simulink model "FOC_beautified"  (R2022b)
settings: Solver=ode1  StartTime=0.0  StopTime=0.2  FixedStep=ctrlConst.TsSwitch  MaxStep=1e-6  RelTol=1e-3  EnableMultiTasking=on
undefined symbols (not defined in the file): ECM, f32_P_AngleCompCur, f32_P_AngleCompVol, f32_P_Coef, f32_P_IdInIF_A, f32_P_Modulation, FFW_enable, g_msgCore0to2_AcrKi, g_msgCore0to2_AcrKiStb, g_msgCore0to2_AcrKp, g_msgCore0to2_AcrKpStb, g_msgCore0to2_AcrSwtHiRpm, g_msgCore0to2_AcrSwtLoRpm, g_msgCore0to2_AfrKp, g_msgCore0to2_AfrTi, g_msgCore0to2_arc_dd_fi, g_msgCore0to2_CalibEn, g_msgCore0to2_clpwitch, g_msgCore0to2_DecoupleEn, g_msgCore0to2_dqLpf, g_msgCore0to2_dqLpfSpdCoef, g_msgCore0to2_FFW_Gain, g_msgCore0to2_linearKpEn, g_msgCore0to2_maxCur, g_msgCore0to2_maxFwcCurRatio, g_msgCore0to2_motorseq, g_msgCore0to2_MTPA_Gain, g_msgCore0to2_pwmFrqSet, g_msgCore0to2_spdswitch, IdROL_C, PWMFrqSwitch_C, SC_Ld_P, SC_Lq_P, SC_Psi_P, Tsw, u16_P_MotorPair
libraries: MathLib x6, simulink x1
(part 1 of 2)
settings Model: Creator=M00039784  LastModifiedBy=HP
settings SolverCC: AlgebraicLoopSolver=TrustRegion  InsertRTBMode=Never (minimum delay)
settings DataIOCC: LimitDataPoints=on  SaveFormat=Array  SaveOutput=off  SaveTime=off
settings OptimizationCC: DefaultParameterBehavior=Inlined  UseDivisionForNetSlopeComputation=on  UseFloatMulNetSlope=on  DefaultUnderspecifiedDataType=single  InlineInvariantSignals=on  PassReuseOutputArgsAs=Individual arguments  ExpressionDepthLimit=2147483647  ZeroExternalMemoryAtStartup=off  ZeroInternalMemoryAtStartup=off  NoFixptDivByZeroProtection=on  EfficientFloat2IntCast=on  LifeSpan=1  EfficientTunableParamExpr=on
settings DebuggingCC: ReadBeforeWriteMsg=DisableAll  WriteAfterWriteMsg=DisableAll  WriteAfterReadMsg=DisableAll  AlgebraicLoopMsg=none  MultiTaskDSMMsg=none  SingleTaskRateTransMsg=error  IntegerOverflowMsg=none  ParameterPrecisionLossMsg=none  FcnCallInpInsideContextMsg=warning  BusObjectLabelMismatch=none  AssertControl=DisableAll  AllowSymbolicDim=off  StateNameClashWarn=warning  SFUnexpectedBacktrackingDiag=warning  SFNoUnconditionalDefaultTransitionDiag=warning  SFExecutionAtInitializationDiag=none  SFMachineParentedDataDiag=warning  IntegerSaturationMsg=none  UnitsInconsistencyMsg=none  ArithmeticOperatorsInVariantConditions=warning
settings HardwareCC: ProdBitPerPointer=32  ProdBitPerSizeT=32  ProdBitPerPtrDiffT=32  ProdLargestAtomicFloat=None  ProdWordSize=32  ProdHWDeviceType=Infineon->TriCore
settings ModelReferenceCC: UpdateModelReferenceTargets=IfOutOfDate  EnableRefExpFcnMdlSchedulingChecks=on  ModelReferenceNumInstancesAllowed=Single  PropagateSignalLabelsOutOfModel=off
settings SFSimCC: SFSimEcho=off  SimUseLocalCustomCode=off  SimGenImportedTypeDefs=on  MATLABDynamicMemAlloc=off  CustomCodeUndefinedFunction=UseInterfaceOnly
settings RTWCC: Description=Embedded Coder  SystemTargetFile=ert.tlc  GenCodeOnly=on  GenerateMakefile=off  TemplateMakefile=ec_target.tmf  RTWVerbose=off  RTWUseLocalCustomCode=off  CodeExecutionProfiling=on  CodeProfilingSaveOptions=AllData  CodeProfilingInstrumentation=detailed
settings CodeAppCC: ForceParamTrailComments=on  IgnoreCustomStorageClasses=off  IgnoreTestpoints=on  MaxIdLength=64  SimulinkDataObjDesc=on  MATLABFcnDesc=on  CustomSymbolStrGlobalVar=pmsmfoc_rt$N$M  CustomSymbolStrType=pmsmfoc_$N$M  CustomSymbolStrFcn=$N$M$F  CustomSymbolStrFcnArg=$I$N$M  CustomSymbolStrMacro=$N$M  InsertBlockDesc=on  StateflowObjectComments=on  MATLABSourceComments=on  InternalIdentifier=Classic
settings ERTTargetCC: TargetLangStandard=C99 (ISO)  UtilityFuncGeneration=Shared location  MultiwordLength=2048  CombineSignalStateStructs=on  SupportAbsoluteTime=off  SupportNonFinite=off  SupportComplex=off  SupportNonInlinedSFcns=on  RemoveResetFunc=off  ParenthesesLevel=Maximum  GenerateASAP2=on  InlinedParameterPlacement=NonHierarchical  ERTCustomFileTemplate=example_file_process.tlc  EnableDataOwnership=on  ConvertIfToSwitch=off  SuppressUnreachableDefaultCases=off  MemSecPackage=Simulink  MemSecDataConstants=MemConst  MemSecDataParameters=MemConstVolatile
settings ConfigComp: CovMetricSettings=dcmtrzow  CovHTMLOptions=-aTS=1 -bRG=1 -bTC=1 -hTR=0 -nFC=0 -scm=1 -bcm=1 -xEv=0  CovSaveCumulativeToWorkspaceVar=on  CovSaveSingleToWorkspaceVar=on  CovExternalEMLEnable=off  CovSFcnEnable=off
settings SimscapeCC: SimscapeNormalizeSystem=off

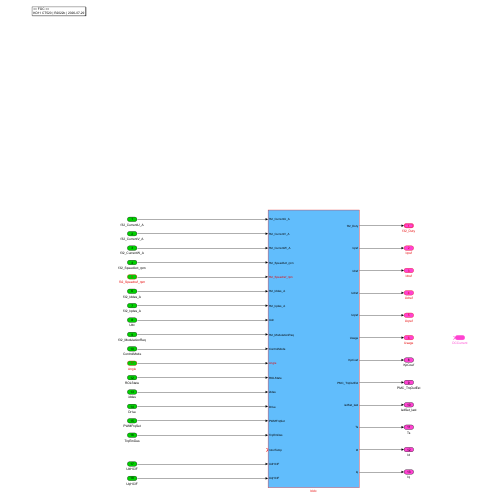
[thumbnail: Simulink's stored preview of the top-level diagram]
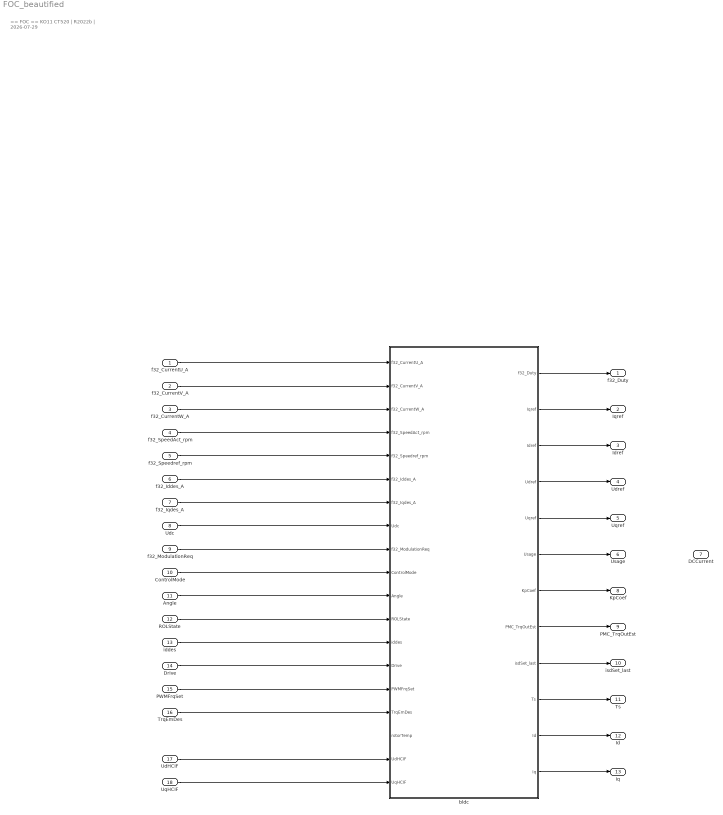
== system FOC_beautified ==
  note: == FOC ==
      | KO11 CT520 | R2022b | 2026-07-29
  f32_CurrentU_A : Inport  OutDataTypeStr=single  PortDimensions=1  SampleTime=0.0001
  f32_CurrentV_A : Inport  Port=2  OutDataTypeStr=single  PortDimensions=1  SampleTime=0.0001
  f32_CurrentW_A : Inport  Port=3  OutDataTypeStr=single  PortDimensions=1  SampleTime=0.0001
  f32_SpeedAct_rpm : Inport  Port=4  OutDataTypeStr=single  PortDimensions=1  SampleTime=0.0001
  f32_Speedref_rpm : Inport  Port=5  OutDataTypeStr=single  PortDimensions=1
  f32_Iddes_A : Inport  Port=6
  f32_Iqdes_A : Inport  Port=7
  "Udc " : Inport  Port=8  OutDataTypeStr=single  PortDimensions=1
  f32_ModulationReq : Inport  Port=9  OutDataTypeStr=single  PortDimensions=1
  ControlMode : Inport  Port=10  OutDataTypeStr=Enum: ECM  PortDimensions=1  SampleTime=0.0001
  Angle : Inport  Port=11  OutDataTypeStr=uint16  PortDimensions=1  SampleTime=0.0001
  ROLState : Inport  Port=12
  iddes : Inport  Port=13
  Drive : Inport  Port=14  OutDataTypeStr=boolean
  PWMFrqSet : Inport  Port=15
  TrqEmDes : Inport  Port=16
  UdHCIF : Inport  Port=17
  UqHCIF : Inport  Port=18
  bldc : Subsystem
  f32_Duty : Outport  OutDataTypeStr=Bus: Duty
  Iqref : Outport  Port=2
  Idref : Outport  Port=3
  Udref : Outport  Port=4
  Uqref : Outport  Port=5
  Usage : Outport  Port=6
  DCCurrent : Outport  Port=7
  KpCoef : Outport  Port=8
  PMC_TrqOutEst : Outport  Port=9
  isdSet_last : Outport  Port=10
  Ts : Outport  Port=11
  Id : Outport  Port=12
  Iq : Outport  Port=13
  wires:
  bldc/6(Usage) -> Usage/1
  f32_Speedref_rpm/1 -> bldc/5(f32_Speedref_rpm)
  f32_Iqdes_A/1 -> bldc/7(f32_Iqdes_A)
  bldc/2(Iqref) -> Iqref/1
  Angle/1 -> bldc/11(Angle)
  bldc/5(Uqref) -> Uqref/1
  f32_CurrentU_A/1 -> bldc/1(f32_CurrentU_A)
  ControlMode/1 -> bldc/10(ControlMode)
  bldc/3(Idref) -> Idref/1
  f32_ModulationReq/1 -> bldc/9(f32_ModulationReq)
  f32_CurrentV_A/1 -> bldc/2(f32_CurrentV_A)
  bldc/1(f32_Duty) -> f32_Duty/1
  f32_SpeedAct_rpm/1 -> bldc/4(f32_SpeedAct_rpm)
  f32_Iddes_A/1 -> bldc/6(f32_Iddes_A)
  f32_CurrentW_A/1 -> bldc/3(f32_CurrentW_A)
  "Udc "/1 -> bldc/8("Udc ")
  bldc/4(Udref) -> Udref/1
  ROLState/1 -> bldc/12(ROLState)
  iddes/1 -> bldc/13(iddes)
  Drive/1 -> bldc/14(Drive)
  PWMFrqSet/1 -> bldc/15(PWMFrqSet)
  bldc/7(KpCoef) -> KpCoef/1
  bldc/8(PMC_TrqOutEst) -> PMC_TrqOutEst/1
  TrqEmDes/1 -> bldc/16(TrqEmDes)
  bldc/9(isdSet_last) -> isdSet_last/1
  bldc/10(Ts) -> Ts/1
  bldc/11(Id) -> Id/1
  bldc/12(Iq) -> Iq/1
  UqHCIF/1 -> bldc/19(UqHCIF)
  UdHCIF/1 -> bldc/18(UdHCIF)

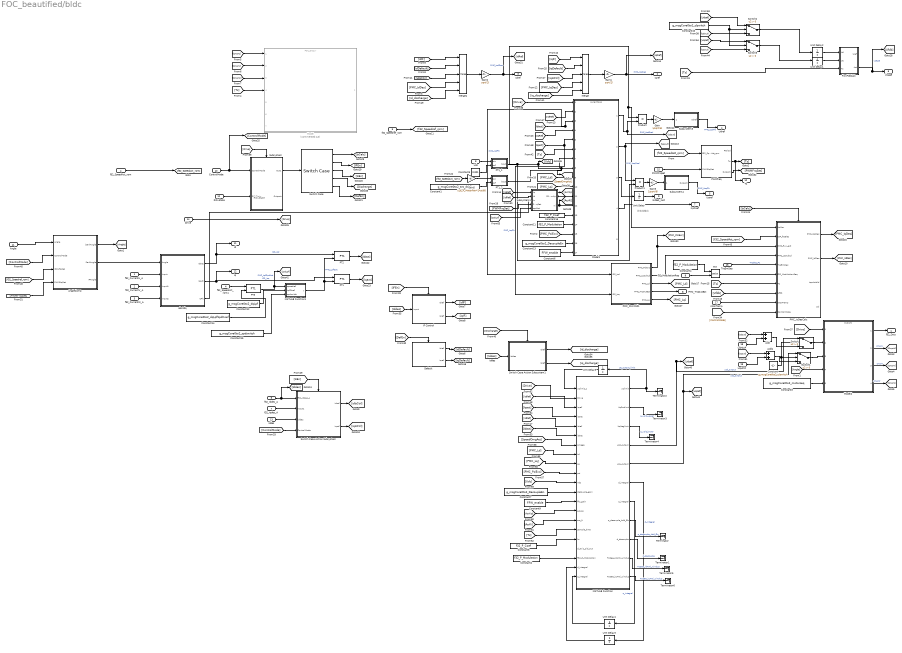
== system FOC_beautified/bldc ==
  note: ROLState
  note: 总电流输出
  f32_CurrentU_A : Inport  OutDataTypeStr=single  PortDimensions=1  SampleTime=0.0001
  f32_CurrentV_A : Inport  Port=2  OutDataTypeStr=single  PortDimensions=1  SampleTime=0.0001
  f32_CurrentW_A : Inport  Port=3  OutDataTypeStr=single  PortDimensions=1  SampleTime=0.0001
  f32_SpeedAct_rpm : Inport  Port=4  OutDataTypeStr=single  PortDimensions=1  SampleTime=0.0001
  f32_Speedref_rpm : Inport  Port=5  OutDataTypeStr=single  PortDimensions=1  SampleTime=0.0001
  f32_Iddes_A : Inport  Port=6
  f32_Iqdes_A : Inport  Port=7
  "Udc " : Inport  Port=8  OutDataTypeStr=single  PortDimensions=1
  f32_ModulationReq : Inport  Port=9
  ControlMode : Inport  Port=10  OutDataTypeStr=Enum: ECM  PortDimensions=1  SampleTime=0.0001
  Angle : Inport  Port=11  OutDataTypeStr=uint16  PortDimensions=1  SampleTime=0.0001
  ROLState : Inport  Port=12
  iddes : Inport  Port=13
  Drive : Inport  Port=14
  PWMFrqSet : Inport  Port=15
  TrqEmDes : Inport  Port=16
  rotorTemp : Inport  Port=17
  UdHCIF : Inport  Port=18
  UqHCIF : Inport  Port=19
  Add : Sum
  Add1 : Sum
  AngleComp : Subsystem  TreatAsAtomicUnit=on
  Constant : Constant  Value=g_msgCore0to2_clpwitch
  Constant1 : Constant  Value=g_msgCore0to2_arc_dd_fi  OutDataTypeStr=single
  Constant10 : Constant  Value=g_msgCore0to2_clpwitch
  Constant11 : Constant  Value=f32_P_Modulation
  Constant12 : Constant  Value=g_msgCore0to2_dqLpf
  Constant13 : Constant  Value=g_msgCore0to2_DecoupleEn
  Constant14 : Constant  Value=g_msgCore0to2_dqLpfSpdCoef
  Constant15 : Constant  Value=g_msgCore0to2_spdswitch
  Constant16 : Constant  Value=f32_P_Coef
  Constant2 : Constant  Value=f32_P_Modulation
  Constant3 : Constant  Value=g_msgCore0to2_motorseq  OutDataTypeStr=uint16
  Constant4 : Constant  Value=f32_P_Modulation  OutDataTypeStr=single
  Constant5 : Constant  Value=0.001  OutDataTypeStr=single
  Constant6 : Constant  Value=FFW_enable
  Constant7 : Constant  Value=g_msgCore0to2_DecoupleEn
  Constant8 : Constant  Value=f32_P_Coef
  Constant9 : Constant  Value=FFW_enable
  Default : Subsystem  TreatAsAtomicUnit=on
  FwcFdbCalc : Subsystem
  Gain : Gain  Gain=1/sqrt(6)
  Gain1 : Gain  Gain=sqrt(2)
  Gain2 : Gain  Gain=sqrt(2)
  Gain3 : Gain  Gain=1/sqrt(6)
  Gain5 : Gain  Gain=u16_P_MotorPair*2*pi/60
  IF Control : Subsystem  TreatAsAtomicUnit=on
  MATLAB Function : MATLAB Function  TreatAsAtomicUnit=on
  MATLAB Function1 : MATLAB Function  TreatAsAtomicUnit=on
  Merge : Merge  Inputs=5  InitialOutput=0
  Merge1 : Merge  Inputs=5  InitialOutput=0
  Min : MinMax  Inputs=2
  Model : ModelReference  Commented=on  ModelNameDialog=FOC_DCCur.slx  SimulationMode=Normal  ModelReferenceVersion=1.22
  Model1 : ModelReference  ModelNameDialog=currentloop.slxp  ModelReferenceVersion=1.125  CopyOfModelProtected=on
  Model2 : ModelReference  ModelNameDialog=SVPWM.slxp  ModelReferenceVersion=1.116  CopyOfModelProtected=on
  PMC_IsDesCalc : Subsystem
  PMC_PsmMdl1 : Subsystem
  PT1 : MathLib/PT1  SystemSampleTime=-1  VariantActivationTime=update diagram  Latency=0  AutoFrameSizeCalculation=off
  PT1_1 : Subsystem
  PT1_2 : Subsystem
  PT2 : MathLib/PT1  SystemSampleTime=-1  VariantActivationTime=update diagram  Latency=0  AutoFrameSizeCalculation=off
  PT3 : MathLib/PT1  SystemSampleTime=-1  VariantActivationTime=update diagram  Latency=0  AutoFrameSizeCalculation=off
  PWMfreq : Subsystem
  Product : Product
  Product1 : Product
  Subsystem : Subsystem
  Subsystem1 : Subsystem
  Subsystem3 : Subsystem
  Subsystem4 : Subsystem
  Switch{,1..3} (4 alike) : Switch  Criteria=u2 > Threshold  SaturateOnIntegerOverflow=off  InputSameDT=off
  Switch Case : SwitchCase  CaseConditions={[ECM.nCtrl,ECM.TrqCtrl],ECM.IFCtrl,[ECM.IsCtrl,ECM.alOfsCal],ECM.Discharge}
  Switch Case Action Subsystem : Subsystem  TreatAsAtomicUnit=on
  Switch Case Action Subsystem1 : Subsystem  TreatAsAtomicUnit=on
  Terminator{,1..6} (7 alike) : Terminator
  Unit Delay{,1..5} (6 alike) : UnitDelay  SampleTime=-1  HasFrameUpgradeWarning=on
  abc2dq : Subsystem
  f32_SpeedAct_rpm1 : InportShadow  Port=4  OutDataTypeStr=single  PortDimensions=1  SampleTime=0.0001
  f32_Duty : Outport  OutDataTypeStr=Bus: Duty
  Iqref : Outport  Port=2
  Idref : Outport  Port=3
  Udref : Outport  Port=4
  Uqref : Outport  Port=5
  Usage : Outport  Port=6
  KpCoef : Outport  Port=7
  PMC_TrqOutEst : Outport  Port=8
  isdSet_last : Outport  Port=9
  Ts : Outport  Port=10
  Id : Outport  Port=11
  Iq : Outport  Port=12
  wires:
  Model2/1 -> f32_Duty/1
  Model1/1 -> Product/2, [Udout]  "PMC_UsdScal"
  f32_SpeedAct_rpm/1 -> [f32_SpeedAct_rpm]
  Model1/2 -> Product1/1, [Uqout]  "PMC_UsqScal"
  PWMfreq/2(Ts) -> Ts/1, [Ts]
  [f32_SpeedAct_rpm] -> PWMfreq/1(f32_SpeedAct_rpm)
  ControlMode/1 -> [ControlMode], Subsystem/1(ControlMode)
  AngleComp/1(iparkAngle) -> [Angle]
  [Idact] -> Model1/3, PMC_PsmMdl1/1(ISP_Isd)  "PMC_isdFlt"
  PT1_1/1(bout) -> Product/1, PMC_IsDesCalc/1(UsMax), [Udc], Model1/7, Product1/2
  [Iqact] -> PMC_PsmMdl1/2(ISP_Isq), Model1/5  "PMC_isqFlt"
  [Ts] -> Model/4
  Model2/2 -> [CmprU]  "cmprU"
  Model2/3 -> [CmprV]  "cmprV"
  Model2/4 -> [CmprW]  "cmprW"
  [CmprW] -> Model/3
  [CmprV] -> Model/2
  [CmprU] -> Model/1
  f32_Iddes_A/1 -> [Iddes], Switch Case Action Subsystem/1(f32_Iddes_A)
  f32_Iqdes_A/1 -> Switch Case Action Subsystem/2(Input1)
  Default/1("Idref ") -> [idDefault]
  [idDefault] -> Merge1/2
  IF Control/1(Idref) -> [idIF]
  [idIF] -> Merge1/1
  IF Control/2(Iqref) -> [iqIF]
  Switch Case Action Subsystem/1("Idref ") -> [idIsCtrl]
  [idIsCtrl] -> Merge1/3
  Merge/1 -> Gain1/1
  [IqRef] -> Model1/4
  Default/2(Iqref) -> [iqDefault]
  Switch Case Action Subsystem/2(Iqref) -> [iqIsCtrl]
  [IFEn] -> IF Control/Action
  Switch Case/2 -> [IFEn]
  [IsEn] -> Switch Case Action Subsystem/Action
  Switch Case/3 -> [IsEn]
  Switch Case/5 -> [DefEn]
  [DefEn] -> Default/Action
  Subsystem/1(Out1) -> Switch Case/1
  ROLState/1 -> Subsystem/2(ROLState)
  iddes/1 -> Switch Case Action Subsystem/3(iddes)
  [ControlMode] -> Switch Case Action Subsystem/4(ControlMode)
  [Iddes] -> IF Control/1(Input)
  Drive/1 -> [Drive]
  [Drive] -> Model1/1
  [Drive] -> Model2/1
  [f32_SpeedAct_rpm] -> Gain5/1
  [Drive] -> Subsystem/Enable
  Model1/3 -> Unit Delay/1
  Unit Delay/1 -> isdSet_last/1
  [Ts] -> Model1/6
  PWMFrqSet/1 -> PWMfreq/2(PWMFrqSet)
  Gain1/1 -> [IqRef], Iqref/1  "PMC_IsqDes"
  Model1/4 -> KpCoef/1
  Product/1 -> Gain/1
  Product1/1 -> Gain3/1
  Subsystem4/1(Outport) -> Uqref/1  "PMC_UsqFlt"
  Gain/1 -> Subsystem3/1(" ")
  Subsystem3/1(Udref) -> Udref/1  "PMC_UsdFlt"
  Gain3/1 -> Subsystem4/1(" ")
  PMC_PsmMdl1/1(PMC_PsiExc) -> [PMC_PsiExc], PMC_IsDesCalc/3(PMC_flux_act)
  PMC_PsmMdl1/2(PMC_LqSubLd) -> PMC_IsDesCalc/4(PMC_LqSubLd)
  PMC_PsmMdl1/4(PMC_TrqOutEst) -> PMC_TrqOutEst/1
  Merge1/1 -> Gain2/1
  Gain2/1 -> [IdRef], Idref/1  "PMC_IsdDes"
  [IdRef] -> Model1/2
  [f32_SpeedAct_rpm] -> PMC_IsDesCalc/2(ISP_frqElec)
  PMC_IsDesCalc/1(PMC_IsqDes) -> [PMC_IqDes]
  TrqEmDes/1 -> PMC_IsDesCalc/5(TrqEmDes)  "Trqdes_P1"
  [iqIF] -> Merge/1
  [iqDefault] -> Merge/2
  [iqIsCtrl] -> Merge/3
  [PMC_IdDes] -> Merge1/4
  [PMC_IqDes] -> Merge/4
  Switch Case/1 -> [IsCalc]
  [IsCalc] -> PMC_IsDesCalc/Action
  PMC_IsDesCalc/2(PMC_IdDes) -> [PMC_IdDes]
  FwcFdbCalc/2(Act) -> [Ufdb], Usage/1  "usage"
  [Ts] -> PMC_IsDesCalc/7(Ts)
  f32_ModulationReq/1 -> Min/2
  f32_CurrentU_A/1 -> abc2dq/2(Input)
  f32_CurrentV_A/1 -> abc2dq/3(Input1)
  f32_CurrentW_A/1 -> abc2dq/4(Input2)
  AngleComp/2(ParkAngle) -> abc2dq/1(Angle)
  [ControlMode] -> AngleComp/2(ControlMode)
  f32_Speedref_rpm/1 -> [f32_Speedref_rpm]
  [f32_Speedref_rpm] -> AngleComp/3(ISP_frqdes)
  abc2dq/1(Idact) -> Id/1, PT2/1  "ISP_isd"
  abc2dq/2(Iqact) -> Iq/1, PT1/1  "ISP_isq"
  Angle/1 -> AngleComp/1(Angle)
  "Udc "/1 -> PT1_1/1(bin)
  Constant5/1 -> PT1_1/2(cof)
  Constant16/1 -> Model1/13
  Constant11/1 -> Model1/14
  [PMC_PsiExc] -> Model1/15
  Constant13/1 -> Model1/16
  Constant6/1 -> Model1/17
  Gain5/1 -> PT1_2/1(bin)
  Constant1/1 -> PT1_2/2(cof)
  PT1_2/1(bout) -> [SpeedOmgAct], Model1/8
  Subsystem1/1(FOC_CurKp) -> Model1/11, [AcrKp]
  Subsystem1/2(Ki) -> [AcrKi], Model1/12
  [IdRef] -> Subsystem1/2(Id)
  [IqRef] -> Subsystem1/1(Iq)
  abc2dq/3(IsFlt) -> Subsystem1/3(Is)
  PMC_PsmMdl1/3(PMC_Ld) -> [PMC_Ld]
  PMC_PsmMdl1/5(PMC_Lq) -> [PMC_Lq]
  [PMC_Ld] -> Model1/9
  [PMC_Lq] -> Model1/10
  Min/1 -> PMC_IsDesCalc/6(f32_ModulationReq)
  Constant4/1 -> Min/1
  [ControlMode] -> PMC_IsDesCalc/10(ControlMode)
  [Ufdb] -> PMC_IsDesCalc/8(Ufdb)
  rotorTemp/1 -> PMC_IsDesCalc/9(rotorTemp)
  Unit Delay1/1 -> FwcFdbCalc/2(Uq)
  Unit Delay2/1 -> FwcFdbCalc/1(Ud)
  [Ts] -> FwcFdbCalc/3(Ts)
  [PWMFrqSet] -> Subsystem1/4(PWMFrqSet)
  PWMfreq/3(Outport) -> [PWMFrqSet]
  [PWMFrqSet] -> AngleComp/4(PWMFrqSet)
  Constant3/1 -> Model2/5
  [Angle] -> Model2/4
  Switch Case/4 -> [Discharge]
  [iq_discharge] -> Merge/5
  [id_discharge] -> Merge1/5
  [Discharge] -> Switch Case Action Subsystem1/Action
  Switch Case Action Subsystem1/1(Idref) -> [id_discharge]
  Switch Case Action Subsystem1/2(Iqref) -> [iq_discharge]
  [Iddes] -> Switch Case Action Subsystem1/1(Iddes)
  [Udout] -> Add/1
  [Uqout] -> Add1/1
  UdHCIF/1 -> Add/2
  UqHCIF/1 -> Add1/2
  [IdRef] -> MATLAB Function/5(idref)
  [Idact] -> MATLAB Function/6(idact)
  [IqRef] -> MATLAB Function/3(iqref)
  [Iqact] -> MATLAB Function/4(iqact)
  [PMC_Ld] -> MATLAB Function/8(Ld)
  [PMC_Lq] -> MATLAB Function/9(Lq)
  [Ts] -> MATLAB Function/16(sample_time)
  Constant7/1 -> MATLAB Function/12(decouple_gain)
  [PMC_PsiExc] -> MATLAB Function/10(psi)
  Constant8/1 -> MATLAB Function/17(kc)
  [SpeedOmgAct] -> MATLAB Function/7(omega)
  [Udc] -> MATLAB Function/11(Vdc)
  [AcrKp] -> MATLAB Function/14(acr_kp)
  [AcrKi] -> MATLAB Function/15(acr_ki)
  Switch/1 -> Model2/2
  Add/1 -> Switch/3
  Switch1/1 -> Model2/3
  Add1/1 -> Switch1/3
  Constant/1 -> Switch1/2, Switch/2
  Unit Delay3/1 -> MATLAB Function/20("d_integral ")
  MATLAB Function/6(d_integral) -> Unit Delay3/1  "d_integral"
  Unit Delay4/1 -> MATLAB Function/21("q_integral ")
  MATLAB Function/7(q_integral) -> Unit Delay4/1  "q_integral"
  MATLAB Function/4(usd_output) -> Switch/1, [Udsef]  "usd_output"
  MATLAB Function/5(usq_output) -> Switch1/1, [Uqsef]  "usq_output"
  [Drive] -> MATLAB Function/2(Drive)
  MATLAB Function/8(q_decouple_Add_ffw) -> Terminator/1  "q_decouple_Add_ffw"
  MATLAB Function/9(d_decouple) -> Terminator1/1  "d_decouple"
  Constant9/1 -> MATLAB Function/13(ffw_gain)
  Constant10/1 -> Switch3/2, Switch2/2
  Switch3/1 -> Unit Delay1/1
  Switch2/1 -> Unit Delay2/1
  MATLAB Function/1(uqlimit) -> Unit Delay5/1, Terminator2/1  "Uq_output_limit"
  [Udout] -> Switch2/3
  [Udsef] -> Switch2/1
  [Uqsef] -> Switch3/1
  [Uqout] -> Switch3/3
  Unit Delay5/1 -> MATLAB Function/1(uqlimit_1)
  MATLAB Function/2(UqPoslimt) -> Terminator3/1  "q_volt_upper"
  MATLAB Function/3(UqNeglimt) -> Terminator4/1  "q_volt_lower"
  Constant2/1 -> MATLAB Function/19(f32_P_Modulation)
  MATLAB Function/10(ToSee_idAnti_windup) -> Terminator5/1  "ToSee_idAnti_windup"
  MATLAB Function/11(ToSee_iqAnti_windup) -> Terminator6/1  "ToSee_iqAnti_windup"
  PT1/1 -> [Iqact]
  PT2/1 -> [Idact]
  MATLAB Function1/1(y) -> PT2/2, PT1/2  "PMC_LpfOpt"
  Constant12/1 -> MATLAB Function1/2(LpfCoef)
  PT3/1 -> [spdLpf], MATLAB Function1/1(speedref)  "PMC_LpfSpdAct"
  f32_SpeedAct_rpm1/1 -> PT3/1
  Constant14/1 -> PT3/2
  [spdLpf] -> Subsystem1/5(spdAct)
  Constant15/1 -> MATLAB Function1/3(spdswitch)

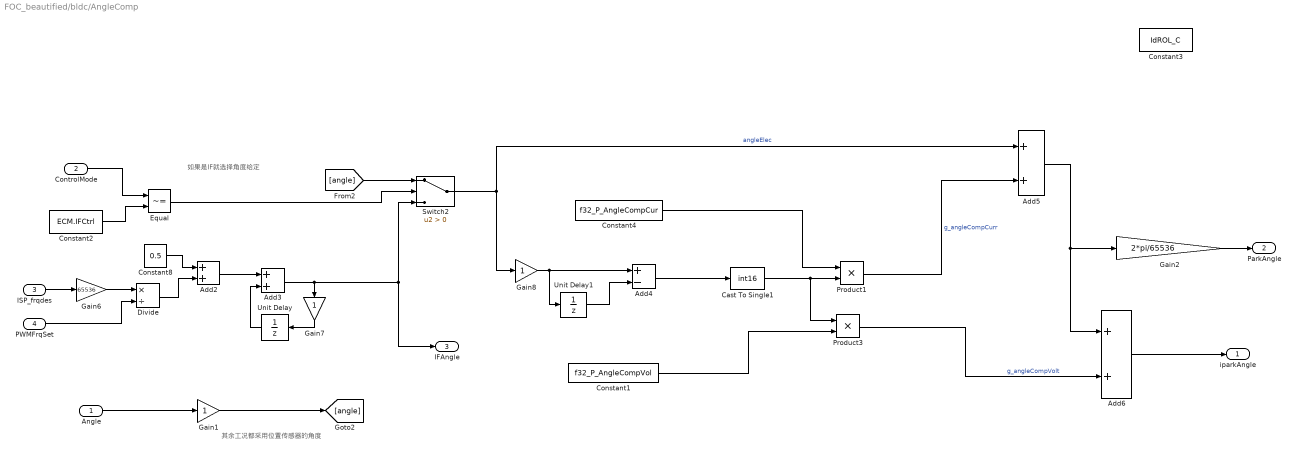
== system FOC_beautified/bldc/AngleComp ==
  note: 如果是IF就选择角度给定
  note: 其余工况都采用位置传感器的角度
  Angle : Inport
  ControlMode : Inport  Port=2
  ISP_frqdes : Inport  Port=3
  PWMFrqSet : Inport  Port=4
  Add2 : Sum  OutDataTypeStr=uint16
  Add3 : Sum
  Add4 : Sum  Inputs=+-  AccumDataTypeStr=int16
  Add5 : Sum  OutDataTypeStr=uint16
  Add6 : Sum  AccumDataTypeStr=uint16  OutDataTypeStr=uint16
  Cast To Single1 : DataTypeConversion  OutDataTypeStr=int16  SaturateOnIntegerOverflow=off  RndMeth=Floor
  Constant1 : Constant  Value=f32_P_AngleCompVol
  Constant2 : Constant  Value=ECM.IFCtrl  OutDataTypeStr=Enum: ECM
  Constant3 : Constant  Value=IdROL_C
  Constant4 : Constant  Value=f32_P_AngleCompCur
  Constant8 : Constant  Value=0.5  OutDataTypeStr=single
  Divide : Product  Inputs=*/
  Equal : RelationalOperator  Operator=~=  OutDataTypeStr=boolean  RndMeth=Simplest  InputSameDT=off
  Gain1 : Gain  OutDataTypeStr=uint16
  Gain2 : Gain  Gain=2*pi/65536  OutDataTypeStr=single
  Gain6 : Gain  Gain=65536
  Gain7 : Gain  OutDataTypeStr=uint16
  Gain8 : Gain  OutDataTypeStr=uint16
  Product1 : Product  OutDataTypeStr=int16
  Product3 : Product  OutDataTypeStr=int16
  Switch2 : Switch  Criteria=u2 > Threshold  SaturateOnIntegerOverflow=off  InputSameDT=off
  Unit Delay : UnitDelay  SampleTime=-1  HasFrameUpgradeWarning=on
  Unit Delay1 : UnitDelay  SampleTime=-1  HasFrameUpgradeWarning=on
  iparkAngle : Outport
  ParkAngle : Outport  Port=2  OutDataTypeStr=single
  IFAngle : Outport  Port=3
  wires:
  Constant2/1 -> Equal/2
  Cast To Single1/1 -> Product3/1, Product1/2
  Product3/1 -> Add6/2  "g_angleCompVolt"
  Constant1/1 -> Product3/2
  Switch2/1 -> Gain8/1, Add5/1  "angleElec"
  Gain8/1 -> Unit Delay1/1, Add4/1
  Constant4/1 -> Product1/1
  Add6/1 -> iparkAngle/1
  Product1/1 -> Add5/2  "g_angleCompCurr"
  Add5/1 -> Add6/1, Gain2/1
  Gain2/1 -> ParkAngle/1
  Add3/1 -> IFAngle/1, Switch2/3, Gain7/1
  Gain7/1 -> Unit Delay/1
  Angle/1 -> Gain1/1
  Unit Delay1/1 -> Add4/2
  Add4/1 -> Cast To Single1/1
  ControlMode/1 -> Equal/1
  [angle] -> Switch2/1
  ISP_frqdes/1 -> Gain6/1
  Add2/1 -> Add3/1
  Gain1/1 -> [angle]
  Unit Delay/1 -> Add3/2
  Equal/1 -> Switch2/2
  Divide/1 -> Add2/2
  Constant8/1 -> Add2/1
  Gain6/1 -> Divide/1
  PWMFrqSet/1 -> Divide/2

== system FOC_beautified/bldc/Default ==
  Action Port : ActionPort  InitializeStates=reset  ActionPortLabel=default:
  Constant : Constant  Value=0  OutDataTypeStr=single
  Constant1 : Constant  Value=0  OutDataTypeStr=single
  "Idref " : Outport  VectorParamsAs1DForOutWhenUnconnected=off
  Iqref : Outport  Port=2  VectorParamsAs1DForOutWhenUnconnected=off
  wires:
  Constant1/1 -> Iqref/1
  Constant/1 -> "Idref "/1

== system FOC_beautified/bldc/FwcFdbCalc ==
  Ud : Inport
  Uq : Inport  Port=2
  Ts : Inport  Port=3
  Add : Sum
  Constant1 : Constant  Value=500  OutDataTypeStr=single
  PT1_1 : Subsystem
  Product : Product  OutDataTypeStr=single
  Product1 : Product  OutDataTypeStr=single
  Product2 : Product
  Sqrt : Sqrt
  Uref : Outport
  Act : Outport  Port=2  VectorParamsAs1DForOutWhenUnconnected=off
  wires:
  Uq/1 -> Product1/2, Product1/1
  Add/1 -> Sqrt/1
  Product1/1 -> Add/2
  Ud/1 -> Product/2, Product/1
  Product/1 -> Add/1
  Sqrt/1 -> Uref/1, PT1_1/1(bin)
  PT1_1/1(bout) -> Act/1
  Product2/1 -> PT1_1/2(cof)
  Constant1/1 -> Product2/2
  Ts/1 -> Product2/1

== system FOC_beautified/bldc/IF Control ==
  Input : Inport
  Action Port : ActionPort  InitializeStates=reset  ActionPortLabel=case [ IFCtrl ]:
  Constant : Constant  Value=f32_P_IdInIF_A  OutDataTypeStr=single
  Constant1 : Constant  Value=0  OutDataTypeStr=single
  Idref : Outport  InitialOutput=0  VectorParamsAs1DForOutWhenUnconnected=off
  Iqref : Outport  Port=2  InitialOutput=0
  wires:
  Input/1 -> Idref/1
  Constant1/1 -> Iqref/1

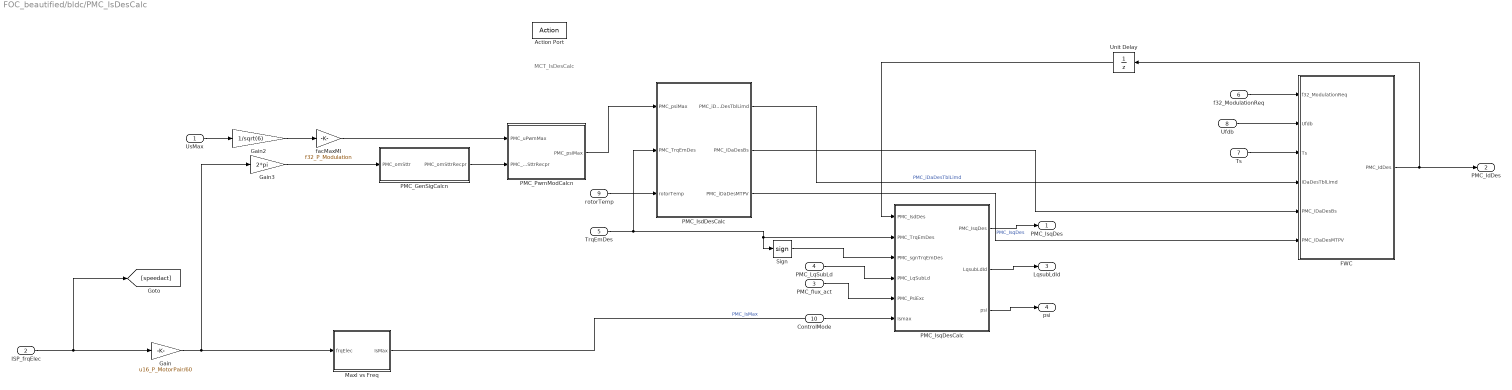
== system FOC_beautified/bldc/PMC_IsDesCalc ==
  note: MCT_IsDesCalc
  UsMax : Inport
  ISP_frqElec : Inport  Port=2
  PMC_flux_act : Inport  Port=3
  PMC_LqSubLd : Inport  Port=4
  TrqEmDes : Inport  Port=5
  f32_ModulationReq : Inport  Port=6  OutDataTypeStr=single  PortDimensions=1
  Ts : Inport  Port=7
  Ufdb : Inport  Port=8
  rotorTemp : Inport  Port=9
  ControlMode : Inport  Port=10
  Action Port : ActionPort  InitializeStates=reset  ActionPortLabel=case [ nCtrl TrqCtrl ]:
  FWC : Subsystem
  Gain : Gain  Gain=u16_P_MotorPair/60
  Gain2 : Gain  Gain=1/sqrt(6)
  Gain3 : Gain  Gain=2*pi
  MaxI vs Freq : Subsystem
  PMC_GenSigCalcn : Subsystem  TreatAsAtomicUnit=on  SystemSampleTime=Tsw
  PMC_IsdDesCalc : Subsystem  TreatAsAtomicUnit=on  SystemSampleTime=Tsw
  PMC_IsqDesCalc : Subsystem  TreatAsAtomicUnit=on  SystemSampleTime=Tsw
  PMC_PwmModCalcn : Subsystem  TreatAsAtomicUnit=on  SystemSampleTime=Tsw
  Sign : Signum
  Unit Delay : UnitDelay  SampleTime=-1  HasFrameUpgradeWarning=on
  facMaxMI : Gain  Gain=f32_P_Modulation  ParamDataTypeStr=single
  PMC_IsqDes : Outport  InitialOutput=0  VectorParamsAs1DForOutWhenUnconnected=off
  PMC_IdDes : Outport  Port=2
  LqsubLdId : Outport  Port=3
  psi : Outport  Port=4
  wires:
  Gain3/1 -> PMC_GenSigCalcn/1(PMC_omSttr)
  PMC_GenSigCalcn/1(PMC_omSttrRecpr) -> PMC_PwmModCalcn/2(PMC_omSttrRecpr)
  facMaxMI/1 -> PMC_PwmModCalcn/1(PMC_uPwmMax)
  PMC_LqSubLd/1 -> PMC_IsqDesCalc/4(PMC_LqSubLd)
  PMC_flux_act/1 -> PMC_IsqDesCalc/5(PMC_PsiExc)
  Sign/1 -> PMC_IsqDesCalc/3(PMC_sgnTrqEmDes)
  TrqEmDes/1 -> PMC_IsdDesCalc/2(PMC_TrqEmDes), Sign/1, PMC_IsqDesCalc/2(PMC_TrqEmDes)
  PMC_PwmModCalcn/1(PMC_psiMax) -> PMC_IsdDesCalc/1(PMC_psiMax)
  Gain/1 -> Gain3/1, MaxI vs Freq/1(frqElec)
  UsMax/1 -> Gain2/1
  ISP_frqElec/1 -> [speedact], Gain/1
  PMC_IsqDesCalc/1(PMC_IsqDes) -> PMC_IsqDes/1  "PMC_IsqDes"
  MaxI vs Freq/1(IsMax) -> PMC_IsqDesCalc/6(Ismax)  "PMC_IsMax"
  PMC_IsdDesCalc/1(PMC_iDaDesTblLimd) -> FWC/4(iDaDesTblLimd)  "PMC_iDaDesTblLimd"
  FWC/1(PMC_IdDes) -> Unit Delay/1, PMC_IdDes/1
  Gain2/1 -> facMaxMI/1
  f32_ModulationReq/1 -> FWC/1(f32_ModulationReq)
  Ufdb/1 -> FWC/2(Ufdb)
  PMC_IsdDesCalc/3(PMC_iDaDesMTPV) -> FWC/6(PMC_iDaDesMTPV)
  Ts/1 -> FWC/3(Ts)
  PMC_IsdDesCalc/2(PMC_iDaDesBs) -> FWC/5(PMC_iDaDesBs)
  Unit Delay/1 -> PMC_IsqDesCalc/1(PMC_IsdDes)
  rotorTemp/1 -> PMC_IsdDesCalc/3(rotorTemp)
  PMC_IsqDesCalc/2(LqsubLdId) -> LqsubLdId/1
  PMC_IsqDesCalc/3(psi) -> psi/1
  ControlMode/1 -> ?

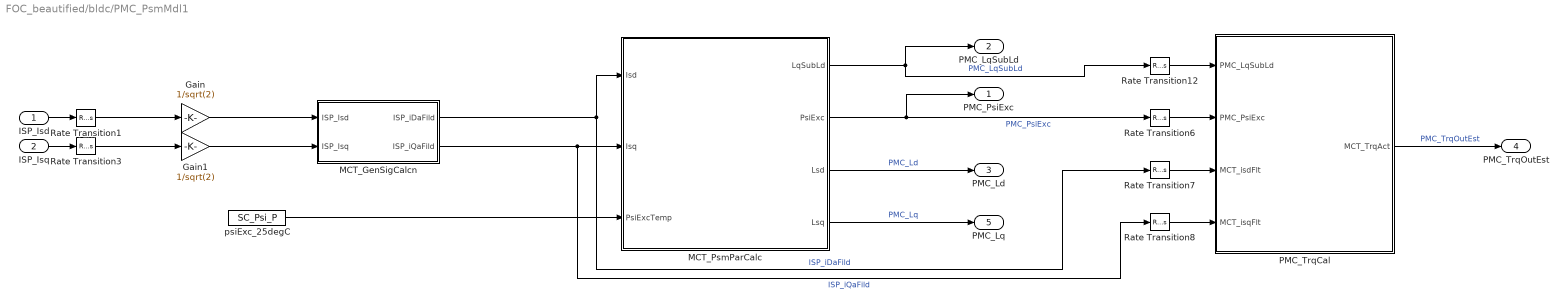
== system FOC_beautified/bldc/PMC_PsmMdl1 ==
  ISP_Isd : Inport
  ISP_Isq : Inport  Port=2
  Gain : Gain  Gain=1/sqrt(2)
  Gain1 : Gain  Gain=1/sqrt(2)
  MCT_GenSigCalcn : Subsystem
  MCT_PsmParCalc : Subsystem  TreatAsAtomicUnit=on
  PMC_TrqCal : Subsystem
  Rate Transition1 : RateTransition  OutPortSampleTime=Tsw
  Rate Transition{6..8,12} (4 alike) : RateTransition  OutPortSampleTime=Ts_1ms
  Rate Transition3 : RateTransition  OutPortSampleTime=Tsw
  psiExc_25degC : Constant  Value=SC_Psi_P  OutDataTypeStr=single  SampleTime=-1
  PMC_PsiExc : Outport  VectorParamsAs1DForOutWhenUnconnected=off
  PMC_LqSubLd : Outport  Port=2  VectorParamsAs1DForOutWhenUnconnected=off
  PMC_Ld : Outport  Port=3  VectorParamsAs1DForOutWhenUnconnected=off
  PMC_TrqOutEst : Outport  Port=4
  PMC_Lq : Outport  Port=5
  wires:
  MCT_PsmParCalc/1(LqSubLd) -> Rate Transition12/1, PMC_LqSubLd/1  "PMC_LqSubLd"
  MCT_PsmParCalc/2(PsiExc) -> PMC_PsiExc/1, Rate Transition6/1  "PMC_PsiExc"
  Rate Transition3/1 -> Gain1/1
  Rate Transition1/1 -> Gain/1
  MCT_GenSigCalcn/1(ISP_iDaFild) -> MCT_PsmParCalc/1(Isd), Rate Transition7/1  "ISP_iDaFild"
  ISP_Isq/1 -> Rate Transition3/1
  ISP_Isd/1 -> Rate Transition1/1
  MCT_GenSigCalcn/2(ISP_iQaFild) -> Rate Transition8/1, MCT_PsmParCalc/2(Isq)  "ISP_iQaFild"
  MCT_PsmParCalc/3(Lsd) -> PMC_Ld/1  "PMC_Ld"
  MCT_PsmParCalc/4(Lsq) -> PMC_Lq/1  "PMC_Lq"
  psiExc_25degC/1 -> MCT_PsmParCalc/3(PsiExcTemp)
  Rate Transition12/1 -> PMC_TrqCal/1(PMC_LqSubLd)
  Rate Transition6/1 -> PMC_TrqCal/2(PMC_PsiExc)
  Rate Transition7/1 -> PMC_TrqCal/3(MCT_isdFlt)
  Rate Transition8/1 -> PMC_TrqCal/4(MCT_isqFlt)
  PMC_TrqCal/1(MCT_TrqAct) -> PMC_TrqOutEst/1  "PMC_TrqOutEst"
  Gain/1 -> MCT_GenSigCalcn/1(ISP_Isd)
  Gain1/1 -> MCT_GenSigCalcn/2(ISP_Isq)

== system FOC_beautified/bldc/PT1_1 ==
  bin : Inport
  cof : Inport  Port=2
  Constant : Constant  OutDataTypeStr=single
  Product1 : Product  RndMeth=Zero  OutDataTypeStr=Inherit: Same as first input
  Product3 : Product  RndMeth=Zero  OutDataTypeStr=Inherit: Same as first input
  Subtract : Sum  Inputs=-+  OutDataTypeStr=Inherit: Same as first input
  Sum1 : Sum  Inputs=|++  OutDataTypeStr=Inherit: Same as first input
  Unit Delay1 : UnitDelay  SampleTime=-1  HasFrameUpgradeWarning=on
  bout : Outport  VectorParamsAs1DForOutWhenUnconnected=off
  wires:
  Product3/1 -> Sum1/2
  Unit Delay1/1 -> Product3/1
  Product1/1 -> Sum1/1
  bin/1 -> Product1/1
  Constant/1 -> Subtract/2
  cof/1 -> Subtract/1, Product1/2
  Sum1/1 -> bout/1, Unit Delay1/1
  Subtract/1 -> Product3/2

== system FOC_beautified/bldc/PT1_2 ==
  bin : Inport
  cof : Inport  Port=2
  Constant : Constant  OutDataTypeStr=single
  Product1 : Product  RndMeth=Zero  OutDataTypeStr=Inherit: Same as first input
  Product3 : Product  RndMeth=Zero  OutDataTypeStr=Inherit: Same as first input
  Subtract : Sum  Inputs=-+  OutDataTypeStr=Inherit: Same as first input
  Sum1 : Sum  Inputs=|++  OutDataTypeStr=Inherit: Same as first input
  Unit Delay1 : UnitDelay  SampleTime=-1  HasFrameUpgradeWarning=on
  bout : Outport  VectorParamsAs1DForOutWhenUnconnected=off
  wires:
  Subtract/1 -> Product3/2
  Sum1/1 -> Unit Delay1/1, bout/1
  cof/1 -> Product1/2, Subtract/1
  Constant/1 -> Subtract/2
  bin/1 -> Product1/1
  Product1/1 -> Sum1/1
  Unit Delay1/1 -> Product3/1
  Product3/1 -> Sum1/2

== system FOC_beautified/bldc/PWMfreq ==
  f32_SpeedAct_rpm : Inport
  PWMFrqSet : Inport  Port=2
  1-D Lookup Table : Lookup_n-D  Commented=on  NumberOfTableDimensions=1  BreakpointsForDimension1=[0 400 800]  Table=[5000;5000;5000]  InternalRulePriority=Speed  OutDataTypeStr=uint32  RndMeth=Simplest
  Constant : Constant  Value=g_msgCore0to2_pwmFrqSet  OutDataTypeStr=single
  Constant1 : Constant  OutDataTypeStr=single
  Constant2 : Constant  Value=PWMFrqSwitch_C
  Divide : Product  Inputs=*/
  Gain : Gain  Gain=100000000  OutDataTypeStr=uint32
  Switch : Switch  Criteria=u2 > Threshold  SaturateOnIntegerOverflow=off  InputSameDT=off
  Period : Outport  OutDataTypeStr=uint32  VectorParamsAs1DForOutWhenUnconnected=off
  Ts : Outport  Port=2  OutDataTypeStr=single
  Outport : Outport  Port=3
  wires:
  Constant/1 -> Switch/3
  f32_SpeedAct_rpm/1 -> 1-D Lookup Table/1
  Divide/1 -> Gain/1, Ts/1
  Constant1/1 -> Divide/1
  Gain/1 -> Period/1
  PWMFrqSet/1 -> Switch/1
  Switch/1 -> Divide/2, Outport/1  "PMC_pwmfrq"
  Constant2/1 -> Switch/2

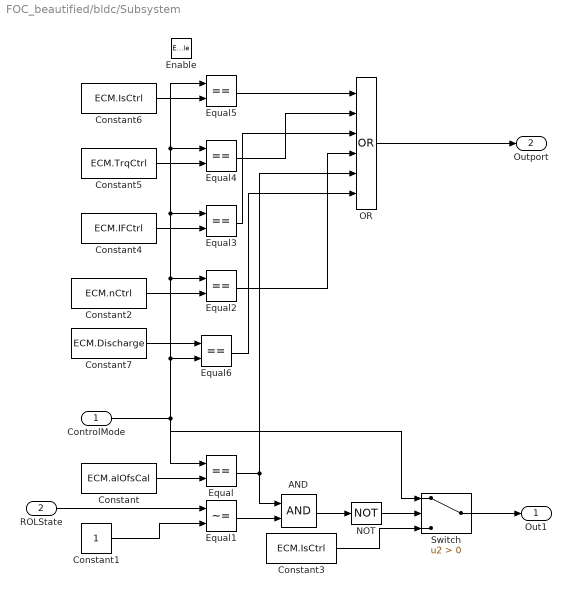
== system FOC_beautified/bldc/Subsystem ==
  ControlMode : Inport
  ROLState : Inport  Port=2
  Enable : EnablePort  StatesWhenEnabling=reset
  AND : Logic  AllPortsSameDT=off  OutDataTypeStr=boolean
  Constant : Constant  Value=ECM.alOfsCal
  Constant1 : Constant  OutDataTypeStr=uint8
  Constant2 : Constant  Value=ECM.nCtrl
  Constant3 : Constant  Value=ECM.IsCtrl
  Constant4 : Constant  Value=ECM.IFCtrl
  Constant5 : Constant  Value=ECM.TrqCtrl
  Constant6 : Constant  Value=ECM.IsCtrl
  Constant7 : Constant  Value=ECM.Discharge
  Equal{,2..6} (6 alike) : RelationalOperator  Operator===  OutDataTypeStr=boolean  RndMeth=Simplest  InputSameDT=off
  Equal1 : RelationalOperator  Operator=~=  OutDataTypeStr=boolean  RndMeth=Simplest  InputSameDT=off
  NOT : Logic  Operator=NOT  IconShape=distinctive  AllPortsSameDT=off  OutDataTypeStr=boolean
  OR : Logic  Operator=OR  Inputs=6  AllPortsSameDT=off  OutDataTypeStr=boolean
  Switch : Switch  Criteria=u2 > Threshold  SaturateOnIntegerOverflow=off  InputSameDT=off
  Out1 : Outport  OutputWhenDisabled=reset  InitialOutput=ECM.Init
  Outport : Outport  Port=2  OutputWhenDisabled=reset  InitialOutput=0
  wires:
  Constant/1 -> Equal/2
  Equal/1 -> OR/5, AND/1
  ROLState/1 -> Equal1/1
  Equal1/1 -> AND/2
  Constant1/1 -> Equal1/2
  AND/1 -> NOT/1
  NOT/1 -> Switch/2
  Switch/1 -> Out1/1
  Constant3/1 -> Switch/3
  Constant2/1 -> Equal2/2
  Constant4/1 -> Equal3/2
  Constant5/1 -> Equal4/2
  Constant6/1 -> Equal5/2
  ControlMode/1 -> Equal6/2, Equal5/1, Equal4/1, Equal3/1, Equal2/1, Equal/1, Switch/1
  Equal5/1 -> OR/1
  Equal4/1 -> OR/2
  Equal3/1 -> OR/3
  Equal2/1 -> OR/4
  OR/1 -> Outport/1
  Constant7/1 -> Equal6/1
  Equal6/1 -> OR/6

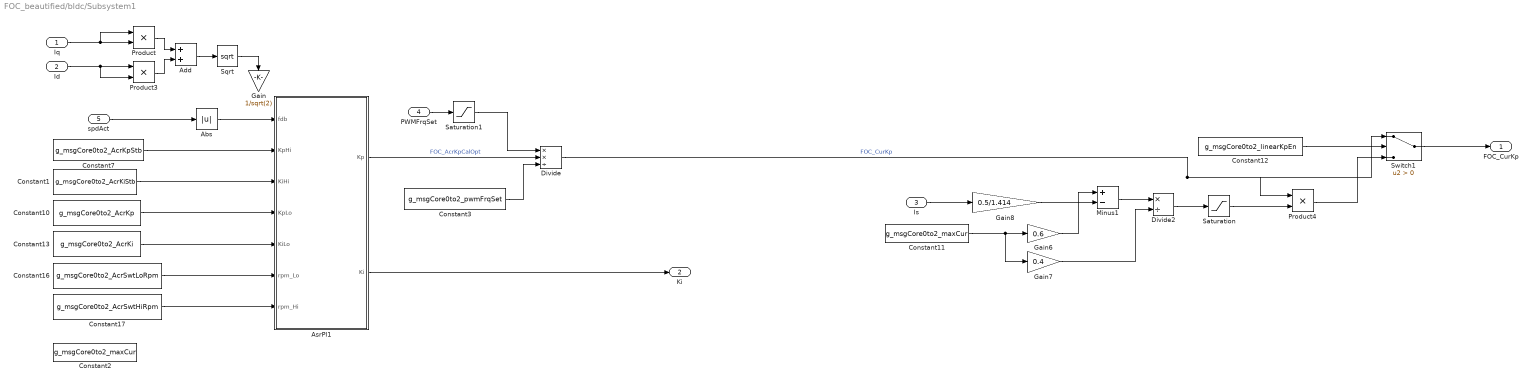
== system FOC_beautified/bldc/Subsystem1 ==
  Iq : Inport
  Id : Inport  Port=2
  Is : Inport  Port=3
  PWMFrqSet : Inport  Port=4
  spdAct : Inport  Port=5
  Abs : Abs  SaturateOnIntegerOverflow=off
  Add : Sum
  AsrPI1 : MATLAB Function
  Constant1 : Constant  Value=g_msgCore0to2_AcrKiStb
  Constant10 : Constant  Value=g_msgCore0to2_AcrKp
  Constant11 : Constant  Value=g_msgCore0to2_maxCur
  Constant12 : Constant  Value=g_msgCore0to2_linearKpEn
  Constant13 : Constant  Value=g_msgCore0to2_AcrKi
  Constant16 : Constant  Value=g_msgCore0to2_AcrSwtLoRpm
  Constant17 : Constant  Value=g_msgCore0to2_AcrSwtHiRpm
  Constant2 : Constant  Value=g_msgCore0to2_maxCur
  Constant3 : Constant  Value=g_msgCore0to2_pwmFrqSet
  Constant7 : Constant  Value=g_msgCore0to2_AcrKpStb
  Divide : Product  Inputs=**/
  Divide2 : Product  Inputs=*/
  Gain : Gain  Gain=1/sqrt(2)
  Gain6 : Gain  Gain=0.6
  Gain7 : Gain  Gain=0.4
  Gain8 : Gain  Gain=0.5/1.414
  Minus1 : Sum  Inputs=+-
  Product : Product
  Product3 : Product
  Product4 : Product
  Saturation : Saturate  UpperLimit=1  LowerLimit=0.5
  Saturation1 : Saturate  UpperLimit=g_msgCore0to2_pwmFrqSet  LowerLimit=2000
  Sqrt : Sqrt
  Switch1 : Switch  Criteria=u2 > Threshold  SaturateOnIntegerOverflow=off  InputSameDT=off
  FOC_CurKp : Outport
  Ki : Outport  Port=2
  wires:
  Gain8/1 -> Minus1/2
  Constant11/1 -> Gain7/1, Gain6/1
  Divide/1 -> Product4/1, Switch1/1  "FOC_CurKp"
  Constant7/1 -> AsrPI1/2(KpHi)
  Minus1/1 -> Divide2/1
  Constant10/1 -> AsrPI1/4(KpLo)
  Constant13/1 -> AsrPI1/5(KiLo)
  Gain7/1 -> Divide2/2
  Constant12/1 -> Switch1/2
  Constant1/1 -> AsrPI1/3(KiHi)
  Divide2/1 -> Saturation/1
  Saturation/1 -> Product4/2
  Switch1/1 -> FOC_CurKp/1
  Gain6/1 -> Minus1/1
  Product4/1 -> Switch1/3
  AsrPI1/2(Ki) -> Ki/1
  Is/1 -> Gain8/1
  Iq/1 -> Product/2, Product/1
  Sqrt/1 -> Gain/1
  Constant16/1 -> AsrPI1/6(rpm_Lo)
  Constant17/1 -> AsrPI1/7(rpm_Hi)
  Id/1 -> Product3/2, Product3/1
  Product/1 -> Add/1
  Product3/1 -> Add/2
  Add/1 -> Sqrt/1
  Constant3/1 -> Divide/3
  PWMFrqSet/1 -> Saturation1/1
  Saturation1/1 -> Divide/1
  AsrPI1/1(Kp) -> Divide/2  "FOC_AcrKpCalOpt"
  spdAct/1 -> Abs/1
  Abs/1 -> AsrPI1/1(fdb)

== system FOC_beautified/bldc/Subsystem3 ==
  " " : Inport
  Constant : Constant  Value=0.1  OutDataTypeStr=single
  Constant1 : Constant  OutDataTypeStr=single
  Minus : Sum  Inputs=+-
  Plus : Sum
  Product : Product
  Product1 : Product
  Unit Delay : UnitDelay  SampleTime=-1  HasFrameUpgradeWarning=on
  Udref : Outport
  wires:
  Plus/1 -> Udref/1, Unit Delay/1
  " "/1 -> Product/2
  Constant/1 -> Minus/2, Product/1
  Minus/1 -> Product1/2
  Product1/1 -> Plus/1
  Constant1/1 -> Minus/1
  Unit Delay/1 -> Product1/1
  Product/1 -> Plus/2

== system FOC_beautified/bldc/Subsystem4 ==
  " " : Inport
  Constant : Constant  Value=0.1  OutDataTypeStr=single
  Constant1 : Constant  OutDataTypeStr=single
  Minus : Sum  Inputs=+-
  Plus : Sum
  Product : Product
  Product1 : Product
  Unit Delay : UnitDelay  SampleTime=-1  HasFrameUpgradeWarning=on
  Outport : Outport
  wires:
  Plus/1 -> Outport/1, Unit Delay/1
  " "/1 -> Product/2
  Constant/1 -> Minus/2, Product/1
  Minus/1 -> Product1/2
  Product1/1 -> Plus/1
  Constant1/1 -> Minus/1
  Unit Delay/1 -> Product1/1
  Product/1 -> Plus/2

== system FOC_beautified/bldc/Switch Case Action Subsystem ==
  f32_Iddes_A : Inport
  Input1 : Inport  Port=2
  iddes : Inport  Port=3
  ControlMode : Inport  Port=4
  Action Port : ActionPort  ActionPortLabel=case [ IsCtrl alOfsCal ]:
  Constant : Constant  Value=ECM.alOfsCal
  Constant1 : Constant  Value=0  OutDataTypeStr=single
  Equal : RelationalOperator  Operator===  OutDataTypeStr=boolean  RndMeth=Simplest  InputSameDT=off
  Switch : Switch  Criteria=u2 > Threshold  SaturateOnIntegerOverflow=off  InputSameDT=off
  Switch1 : Switch  Criteria=u2 > Threshold  SaturateOnIntegerOverflow=off  InputSameDT=off
  "Idref " : Outport  InitialOutput=0  VectorParamsAs1DForOutWhenUnconnected=off
  Iqref : Outport  Port=2  InitialOutput=0  VectorParamsAs1DForOutWhenUnconnected=off
  wires:
  ControlMode/1 -> Equal/1
  Constant/1 -> Equal/2
  Switch/1 -> "Idref "/1
  Switch1/1 -> Iqref/1
  Equal/1 -> Switch1/2, Switch/2
  f32_Iddes_A/1 -> Switch/3
  Input1/1 -> Switch1/3
  iddes/1 -> Switch/1
  Constant1/1 -> Switch1/1

== system FOC_beautified/bldc/Switch Case Action Subsystem1 ==
  Iddes : Inport
  Action Port : ActionPort  InitializeStates=reset  ActionPortLabel=case [ Discharge ]:
  Iqdes : Constant  Value=0  OutDataTypeStr=single
  Idref : Outport  InitialOutput=0  VectorParamsAs1DForOutWhenUnconnected=off
  Iqref : Outport  Port=2  InitialOutput=0
  wires:
  Iqdes/1 -> Iqref/1
  Iddes/1 -> Idref/1

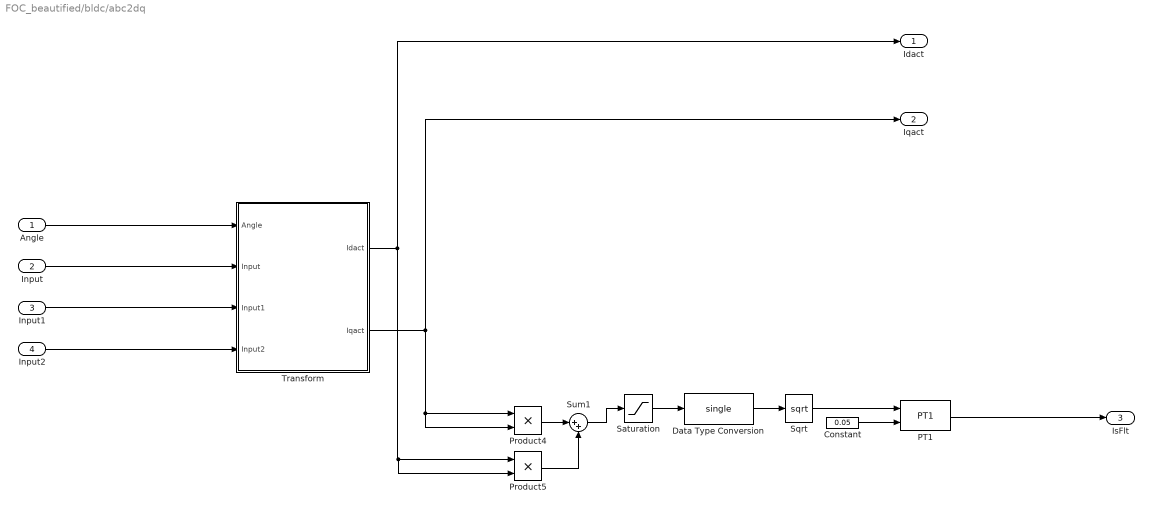
== system FOC_beautified/bldc/abc2dq ==
  Angle : Inport
  Input : Inport  Port=2
  Input1 : Inport  Port=3
  Input2 : Inport  Port=4
  Constant : Constant  Value=0.05  OutDataTypeStr=single
  Data Type Conversion : DataTypeConversion  OutDataTypeStr=single  SaturateOnIntegerOverflow=off  RndMeth=Floor
  PT1 : MathLib/PT1  SystemSampleTime=-1  VariantActivationTime=update diagram  Latency=0  AutoFrameSizeCalculation=off
  Product4 : Product  OutDataTypeStr=Inherit: Inherit via back propagation  RndMeth=Zero
  Product5 : Product  RndMeth=Zero
  Saturation : Saturate  UpperLimit=inf  LowerLimit=0
  Sqrt : Sqrt
  Sum1 : Sum  Priority=25  Inputs=|++
  Transform : Subsystem
  Idact : Outport  VectorParamsAs1DForOutWhenUnconnected=off
  Iqact : Outport  Port=2  VectorParamsAs1DForOutWhenUnconnected=off
  IsFlt : Outport  Port=3  VectorParamsAs1DForOutWhenUnconnected=off
  wires:
  Angle/1 -> Transform/1(Angle)
  Transform/1(Idact) -> Idact/1, Product5/2, Product5/1
  Sqrt/1 -> PT1/1
  Constant/1 -> PT1/2
  Product4/1 -> Sum1/1
  Product5/1 -> Sum1/2
  PT1/1 -> IsFlt/1
  Sum1/1 -> Saturation/1
  Saturation/1 -> Data Type Conversion/1
  Data Type Conversion/1 -> Sqrt/1
  Transform/2(Iqact) -> Iqact/1, Product4/2, Product4/1
  Input/1 -> Transform/2(Input)
  Input1/1 -> Transform/3(Input1)
  Input2/1 -> Transform/4(Input2)

== system FOC_beautified/bldc/FwcFdbCalc/PT1_1 ==
  bin : Inport
  cof : Inport  Port=2
  Constant : Constant  OutDataTypeStr=single
  Product1 : Product  RndMeth=Zero  OutDataTypeStr=Inherit: Same as first input
  Product3 : Product  RndMeth=Zero  OutDataTypeStr=Inherit: Same as first input
  Subtract : Sum  Inputs=-+  OutDataTypeStr=Inherit: Same as first input
  Sum1 : Sum  Inputs=|++  OutDataTypeStr=Inherit: Same as first input
  Unit Delay1 : UnitDelay  SampleTime=-1  HasFrameUpgradeWarning=on
  bout : Outport  VectorParamsAs1DForOutWhenUnconnected=off
  wires:
  Product3/1 -> Sum1/2
  Unit Delay1/1 -> Product3/1
  Product1/1 -> Sum1/1
  bin/1 -> Product1/1
  Constant/1 -> Subtract/2
  cof/1 -> Subtract/1, Product1/2
  Sum1/1 -> bout/1, Unit Delay1/1
  Subtract/1 -> Product3/2

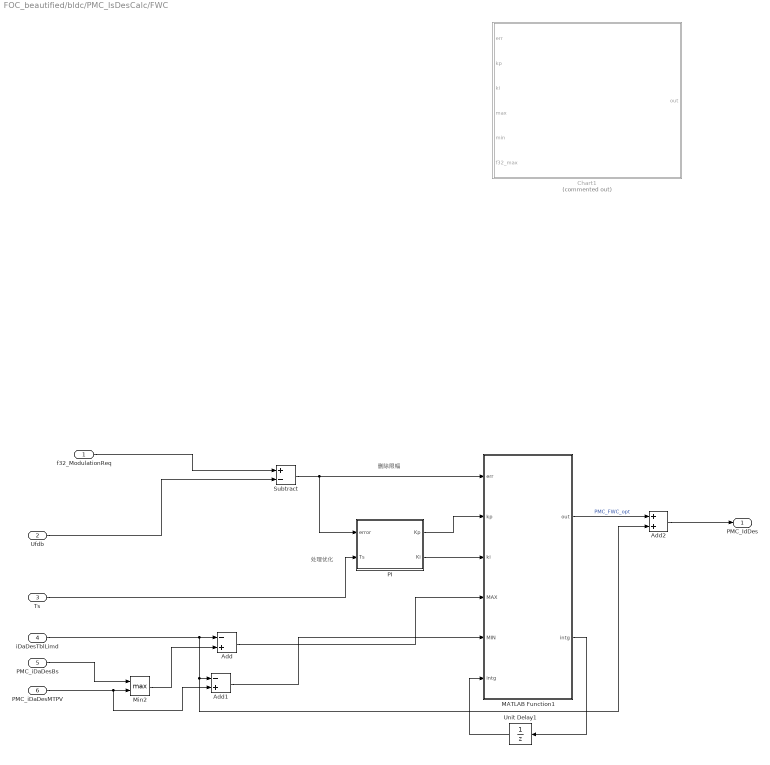
== system FOC_beautified/bldc/PMC_IsDesCalc/FWC ==
  note: 处理优化
  note: 删除限幅
  f32_ModulationReq : Inport
  Ufdb : Inport  Port=2
  Ts : Inport  Port=3
  iDaDesTblLimd : Inport  Port=4
  PMC_iDaDesBs : Inport  Port=5
  PMC_iDaDesMTPV : Inport  Port=6
  Add : Sum  Inputs=-+
  Add1 : Sum  Inputs=-+
  Add2 : Sum
  Chart1 : Stateflow chart  Commented=on  TreatAsAtomicUnit=on
  MATLAB Function1 : MATLAB Function  TreatAsAtomicUnit=on
  Min2 : MinMax  Function=max  Inputs=2
  PI : Subsystem
  Subtract : Sum  Inputs=+-
  Unit Delay1 : UnitDelay  SampleTime=-1  HasFrameUpgradeWarning=on
  PMC_IdDes : Outport  OutputWhenDisabled=reset  InitialOutput=0  VectorParamsAs1DForOutWhenUnconnected=off
  wires:
  PI/1(Kp) -> MATLAB Function1/2(kp)
  Add/1 -> MATLAB Function1/4(MAX)
  Add1/1 -> MATLAB Function1/5(MIN)
  Subtract/1 -> PI/1(error), MATLAB Function1/1(err)
  f32_ModulationReq/1 -> Subtract/1
  Unit Delay1/1 -> MATLAB Function1/6("intg ")
  MATLAB Function1/2(intg) -> Unit Delay1/1
  PI/2(Ki) -> MATLAB Function1/3(ki)
  Ts/1 -> PI/2(Ts)
  PMC_iDaDesBs/1 -> Min2/1
  PMC_iDaDesMTPV/1 -> Add1/2, Min2/2
  Min2/1 -> Add/2
  iDaDesTblLimd/1 -> Add1/1, Add2/2, Add/1
  MATLAB Function1/1(out) -> Add2/1  "PMC_FWC_opt"
  Add2/1 -> PMC_IdDes/1
  Ufdb/1 -> Subtract/2

== system FOC_beautified/bldc/PMC_IsDesCalc/MaxI vs Freq ==
  frqElec : Inport
  Abs : Abs  SaturateOnIntegerOverflow=off
  Freq vs MaxI : Lookup_n-D  NumberOfTableDimensions=1  DataSpecification=Lookup table object  LookupTableObject=facIphaMaxFreq_T  BreakpointsForDimension1=[0 1 5 10 20 50 100 200 300 400 800 1600]  BeginIndexSearchUsingPreviousIndexResult=on  Table=[0.5 0.5 0.6 0.7 0.75 0.8 0.85 0.9 0.97 1 1 1]  ExtrapMethod=Clip  UseLastTableValue=on  InternalRulePriority=Speed  OutDataTypeStr=Inherit: Inherit from 'Table data'
  Ismax1 : Constant  Value=g_msgCore0to2_maxCur  OutDataTypeStr=single
  PT1_2 : Subsystem
  Terminator : Terminator
  tauPT1IsMax : Constant  Value=0.1  OutDataTypeStr=single
  IsMax : Outport  VectorParamsAs1DForOutWhenUnconnected=off
  wires:
  frqElec/1 -> Abs/1
  PT1_2/1(bout) -> Freq vs MaxI/1
  Ismax1/1 -> IsMax/1
  tauPT1IsMax/1 -> PT1_2/2(cof)
  Abs/1 -> PT1_2/1(bin)
  Freq vs MaxI/1 -> Terminator/1

== system FOC_beautified/bldc/PMC_IsDesCalc/PMC_GenSigCalcn ==
  PMC_omSttr : Inport
  Abs : Abs  SaturateOnIntegerOverflow=off
  Divide : Product  Inputs=*/
  MinMax : MinMax  Function=max  Inputs=2
  unit : Constant  OutDataTypeStr=single  SampleTime=-1
  w10Hz : Constant  Value=10*2*pi  OutDataTypeStr=single  SampleTime=-1
  PMC_omSttrRecpr : Outport  SampleTime=Tsw  VectorParamsAs1DForOutWhenUnconnected=off
  wires:
  w10Hz/1 -> MinMax/1
  MinMax/1 -> Divide/2
  Abs/1 -> MinMax/2
  Divide/1 -> PMC_omSttrRecpr/1
  unit/1 -> Divide/1
  PMC_omSttr/1 -> Abs/1

== system FOC_beautified/bldc/PMC_IsDesCalc/PMC_IsdDesCalc ==
  note: 此除参考EP32软件更改
  PMC_psiMax : Inport
  PMC_TrqEmDes : Inport  Port=2
  rotorTemp : Inport  Port=3
  iDaDesTblLimd : Subsystem
  PMC_iDaDesTblLimd : Outport  VectorParamsAs1DForOutWhenUnconnected=off
  PMC_iDaDesBs : Outport  Port=2  VectorParamsAs1DForOutWhenUnconnected=off
  PMC_iDaDesMTPV : Outport  Port=3  VectorParamsAs1DForOutWhenUnconnected=off
  wires:
  iDaDesTblLimd/2(iDaDesTblLimd) -> PMC_iDaDesTblLimd/1
  PMC_TrqEmDes/1 -> iDaDesTblLimd/2(PMC_TrqEmDes)
  PMC_psiMax/1 -> iDaDesTblLimd/1(PMC_psiMax)
  iDaDesTblLimd/3(iDaDesBS) -> PMC_iDaDesBs/1  "BS"
  iDaDesTblLimd/1(iDaDesMTPV) -> PMC_iDaDesMTPV/1  "MTPV"
  rotorTemp/1 -> iDaDesTblLimd/3(rotorTemp)

== system FOC_beautified/bldc/PMC_IsDesCalc/PMC_IsqDesCalc ==
  PMC_IsdDes : Inport
  PMC_TrqEmDes : Inport  Port=2
  PMC_sgnTrqEmDes : Inport  Port=3
  PMC_LqSubLd : Inport  Port=4
  PMC_PsiExc : Inport  Port=5
  Ismax : Inport  Port=6
  Index Vector : MultiPortSwitch  DataPortOrder=Zero-based contiguous  Inputs=2  zeroidx=on  SaturateOnIntegerOverflow=off  InputSameDT=off
  IsqDesLim_Calc : Subsystem  TreatAsAtomicUnit=on
  IsqTrqDes_Calc : Subsystem  TreatAsAtomicUnit=on
  PMC_IsqDes : Outport  VectorParamsAs1DForOutWhenUnconnected=off
  LqsubLdId : Outport  Port=2
  psi : Outport  Port=3
  wires:
  PMC_sgnTrqEmDes/1 -> IsqDesLim_Calc/3(MCT_sgnTrqEmDes)
  IsqTrqDes_Calc/1(IsqTrqDes) -> IsqDesLim_Calc/1(IsqTrqDes), Index Vector/2
  PMC_IsdDes/1 -> IsqTrqDes_Calc/2(MCT_IsdDes), IsqDesLim_Calc/2(MCT_IsdDes)
  PMC_PsiExc/1 -> IsqTrqDes_Calc/4(MCT_PsiExc)
  PMC_LqSubLd/1 -> IsqTrqDes_Calc/3(MCT_LqSubLd)
  PMC_TrqEmDes/1 -> IsqTrqDes_Calc/1(MCT_TrqEmDes)
  IsqDesLim_Calc/2(IsqDesLim) -> Index Vector/3
  IsqDesLim_Calc/1(bIsResLimActv) -> Index Vector/1
  Ismax/1 -> IsqDesLim_Calc/4(Ismax)
  Index Vector/1 -> PMC_IsqDes/1
  IsqTrqDes_Calc/2(LqsubLdId) -> LqsubLdId/1
  IsqTrqDes_Calc/3(psi) -> psi/1

== system FOC_beautified/bldc/PMC_IsDesCalc/PMC_PwmModCalcn ==
  PMC_uPwmMax : Inport
  PMC_omSttrRecpr : Inport  Port=2
  Product : Product  RndMeth=Zero
  PMC_psiMax : Outport  VectorParamsAs1DForOutWhenUnconnected=off
  wires:
  Product/1 -> PMC_psiMax/1
  PMC_omSttrRecpr/1 -> Product/2
  PMC_uPwmMax/1 -> Product/1

== system FOC_beautified/bldc/PMC_PsmMdl1/MCT_GenSigCalcn ==
  ISP_Isd : Inport
  ISP_Isq : Inport  Port=2
  PT1 : MathLib/PT1  SystemSampleTime=-1  VariantActivationTime=update diagram  Latency=0  AutoFrameSizeCalculation=off
  PT2 : MathLib/PT1  SystemSampleTime=-1  VariantActivationTime=update diagram  Latency=0  AutoFrameSizeCalculation=off
  tauPT1Isd : Constant  Value=0.1  OutDataTypeStr=single
  ISP_iDaFild : Outport  VectorParamsAs1DForOutWhenUnconnected=off
  ISP_iQaFild : Outport  Port=2  VectorParamsAs1DForOutWhenUnconnected=off
  wires:
  ISP_Isq/1 -> PT2/1
  PT2/1 -> ISP_iQaFild/1
  tauPT1Isd/1 -> PT2/2, PT1/2
  ISP_Isd/1 -> PT1/1
  PT1/1 -> ISP_iDaFild/1
